simulink model "old_FMS"  (R2018b)
settings: configuration reference "FMS_config" (kept outside this file)
undefined symbols (not defined in the file): actuator_cmd, DiscIntNeverNeededParam, FMS_EXPORT, FMS_PARAM, mode, p_cmd, phi_cmd, psi_rate_cmd, q_cmd, r_cmd, reset, state, theta_cmd, throttle_cmd, timestamp, u_cmd, v_cmd, w_cmd
libraries: simulink x39, Rotation x2, Filter x1
(part 2 of 2)

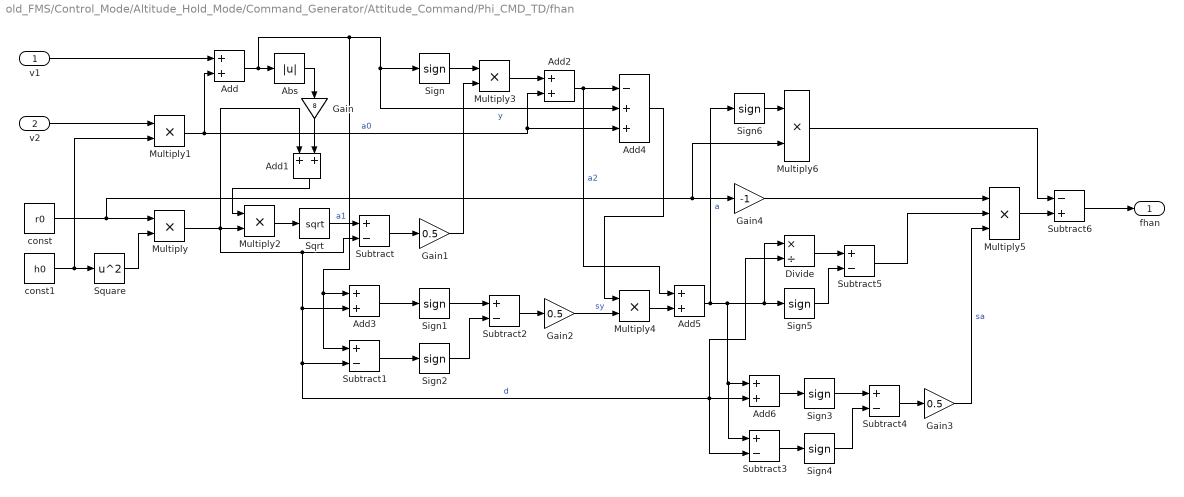
== system old_FMS/Control_Mode/Altitude_Hold_Mode/Command_Generator/Attitude_Command/Phi_CMD_TD/fhan  ==
  v1 : Inport
  v2 : Inport  Port=2
  Abs : Abs
  Add{,1..3,5..6} (6 alike) : Sum  OutDataTypeStr=Inherit: Same as first input
  Add4 : Sum  Inputs=-++
  Divide : Product  Inputs=*/
  Gain : Gain  Gain=8
  Gain1 : Gain  Gain=0.5  OutDataTypeStr=Inherit: Same as input
  Gain2 : Gain  Gain=0.5  OutDataTypeStr=Inherit: Same as input
  Gain3 : Gain  Gain=0.5  OutDataTypeStr=Inherit: Same as input
  Gain4 : Gain  Gain=-1  OutDataTypeStr=Inherit: Same as input
  Multiply{,1..3} (4 alike) : Product  OutDataTypeStr=Inherit: Same as first input
  Multiply4 : Product  OutDataTypeStr=single
  Multiply5 : Product  Inputs=3
  Multiply6 : Product  OutDataTypeStr=single
  Sign{,1..6} (7 alike) : Signum
  Sqrt : Sqrt  SaturateOnIntegerOverflow=on
  Square : Math  Operator=square  SaturateOnIntegerOverflow=on
  Subtract{,1..5} (6 alike) : Sum  Inputs=+-  OutDataTypeStr=Inherit: Same as first input
  Subtract6 : Sum  Inputs=-+  OutDataTypeStr=Inherit: Same as first input
  const : Constant  Value=r0  OutDataTypeStr=single
  const1 : Constant  Value=h0  OutDataTypeStr=single
  fhan : Outport
  wires:
  Sign1/1 -> Subtract2/1
  Multiply2/1 -> Sqrt/1
  Square/1 -> Multiply/2
  Gain1/1 -> Multiply3/2
  Multiply6/1 -> Subtract6/1
  Multiply/1 -> Multiply2/2, Add1/1, Add3/2, Subtract1/2, Add6/2, Subtract3/2, Divide/2, Subtract/2  "d"
  Add6/1 -> Sign3/1
  Sign3/1 -> Subtract4/1
  Sign6/1 -> Multiply6/1
  Multiply5/1 -> Subtract6/2
  Gain4/1 -> Multiply5/1
  Subtract4/1 -> Gain3/1
  Add2/1 -> Add5/1, Add4/1  "a2"
  Subtract2/1 -> Gain2/1
  Add/1 -> Abs/1, Sign/1, Add4/2, Add3/1, Subtract1/1  "y"
  Multiply1/1 -> Add/2, Add2/2, Add4/3  "a0"
  Add5/1 -> Add6/1, Subtract3/1, Divide/1, Sign5/1, Sign6/1  "a"
  const1/1 -> Square/1, Multiply1/2
  Multiply4/1 -> Add5/2
  Subtract5/1 -> Multiply5/2
  Add3/1 -> Sign1/1
  const/1 -> Multiply/1, Gain4/1, Multiply6/2
  Gain/1 -> Add1/2
  Multiply3/1 -> Add2/1
  Divide/1 -> Subtract5/1
  Subtract1/1 -> Sign2/1
  Add1/1 -> Multiply2/1
  Subtract3/1 -> Sign4/1
  Sqrt/1 -> Subtract/1  "a1"
  Sign5/1 -> Subtract5/2
  Add4/1 -> Multiply4/1
  Abs/1 -> Gain/1
  Sign4/1 -> Subtract4/2
  Sign2/1 -> Subtract2/2
  Subtract6/1 -> fhan/1
  Subtract/1 -> Gain1/1
  Gain3/1 -> Multiply5/3  "sa"
  v2/1 -> Multiply1/1
  Gain2/1 -> Multiply4/2  "sy"
  Sign/1 -> Multiply3/1
  v1/1 -> Add/1

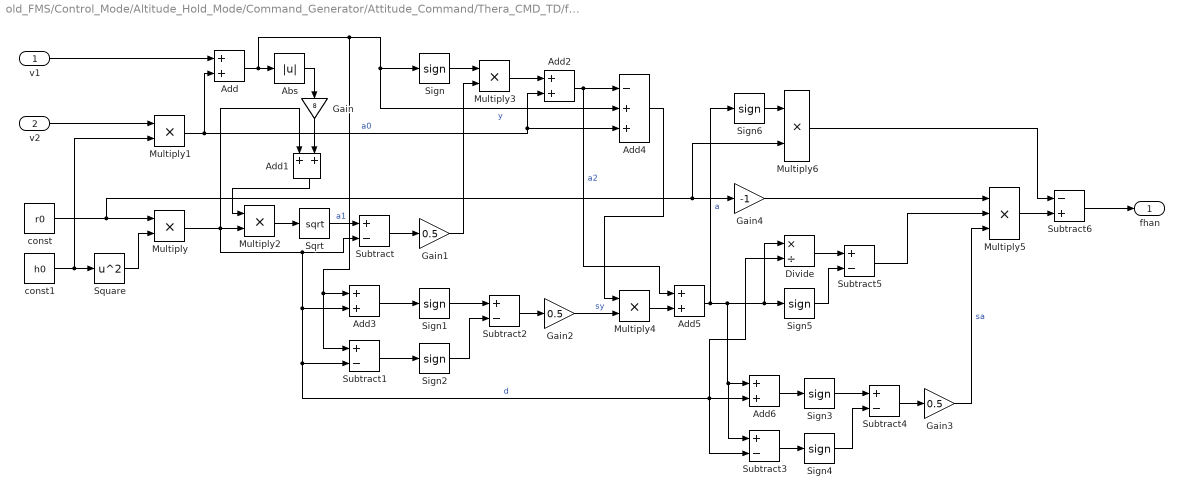
== system old_FMS/Control_Mode/Altitude_Hold_Mode/Command_Generator/Attitude_Command/Thera_CMD_TD/fhan  ==
  v1 : Inport
  v2 : Inport  Port=2
  Abs : Abs
  Add{,1..3,5..6} (6 alike) : Sum  OutDataTypeStr=Inherit: Same as first input
  Add4 : Sum  Inputs=-++
  Divide : Product  Inputs=*/
  Gain : Gain  Gain=8
  Gain1 : Gain  Gain=0.5  OutDataTypeStr=Inherit: Same as input
  Gain2 : Gain  Gain=0.5  OutDataTypeStr=Inherit: Same as input
  Gain3 : Gain  Gain=0.5  OutDataTypeStr=Inherit: Same as input
  Gain4 : Gain  Gain=-1  OutDataTypeStr=Inherit: Same as input
  Multiply{,1..3} (4 alike) : Product  OutDataTypeStr=Inherit: Same as first input
  Multiply4 : Product  OutDataTypeStr=single
  Multiply5 : Product  Inputs=3
  Multiply6 : Product  OutDataTypeStr=single
  Sign{,1..6} (7 alike) : Signum
  Sqrt : Sqrt  SaturateOnIntegerOverflow=on
  Square : Math  Operator=square  SaturateOnIntegerOverflow=on
  Subtract{,1..5} (6 alike) : Sum  Inputs=+-  OutDataTypeStr=Inherit: Same as first input
  Subtract6 : Sum  Inputs=-+  OutDataTypeStr=Inherit: Same as first input
  const : Constant  Value=r0  OutDataTypeStr=single
  const1 : Constant  Value=h0  OutDataTypeStr=single
  fhan : Outport
  wires:
  Sign1/1 -> Subtract2/1
  Multiply2/1 -> Sqrt/1
  Square/1 -> Multiply/2
  Gain1/1 -> Multiply3/2
  Multiply6/1 -> Subtract6/1
  Multiply/1 -> Multiply2/2, Add1/1, Add3/2, Subtract1/2, Add6/2, Subtract3/2, Divide/2, Subtract/2  "d"
  Add6/1 -> Sign3/1
  Sign3/1 -> Subtract4/1
  Sign6/1 -> Multiply6/1
  Multiply5/1 -> Subtract6/2
  Gain4/1 -> Multiply5/1
  Subtract4/1 -> Gain3/1
  Add2/1 -> Add5/1, Add4/1  "a2"
  Subtract2/1 -> Gain2/1
  Add/1 -> Abs/1, Sign/1, Add4/2, Add3/1, Subtract1/1  "y"
  Multiply1/1 -> Add/2, Add2/2, Add4/3  "a0"
  Add5/1 -> Add6/1, Subtract3/1, Divide/1, Sign5/1, Sign6/1  "a"
  const1/1 -> Square/1, Multiply1/2
  Multiply4/1 -> Add5/2
  Subtract5/1 -> Multiply5/2
  Add3/1 -> Sign1/1
  const/1 -> Multiply/1, Gain4/1, Multiply6/2
  Gain/1 -> Add1/2
  Multiply3/1 -> Add2/1
  Divide/1 -> Subtract5/1
  Subtract1/1 -> Sign2/1
  Add1/1 -> Multiply2/1
  Subtract3/1 -> Sign4/1
  Sqrt/1 -> Subtract/1  "a1"
  Sign5/1 -> Subtract5/2
  Add4/1 -> Multiply4/1
  Abs/1 -> Gain/1
  Sign4/1 -> Subtract4/2
  Sign2/1 -> Subtract2/2
  Subtract6/1 -> fhan/1
  Subtract/1 -> Gain1/1
  Gain3/1 -> Multiply5/3  "sa"
  v2/1 -> Multiply1/1
  Gain2/1 -> Multiply4/2  "sy"
  Sign/1 -> Multiply3/1
  v1/1 -> Add/1

== system old_FMS/Control_Mode/Altitude_Hold_Mode/Command_Generator/Psi_Rate_Command/Heading_Control/Heading_Error ==
  INS_Out : Inport
  update : Inport  Port=2
  Bus_Selection : Subsystem
  Holder : Subsystem
  Sum : Sum  Inputs=-+|
  psi_err_rad : Outport
  wires:
  Bus_Selection/1(psi_rad) -> Sum/1, Holder/1(u)
  update/1 -> Holder/2(update)
  INS_Out/1 -> Bus_Selection/1(INS_Out)
  Holder/1(y) -> Sum/2  "psi_hold"
  Sum/1 -> psi_err_rad/1  "psi_err"

== system old_FMS/Control_Mode/Altitude_Hold_Mode/Command_Generator/Psi_Rate_Command/Heading_Rate_Map/Stretch ==
  u : Inport
  Dead Zone : DeadZone  LowerValue=-FMS_PARAM.StickDeadZone  UpperValue=FMS_PARAM.StickDeadZone  SaturateOnIntegerOverflow=on
  Gain : Gain  Gain=1/(1-FMS_PARAM.StickDeadZone)
  y : Outport
  wires:
  u/1 -> Dead Zone/1
  Dead Zone/1 -> Gain/1
  Gain/1 -> y/1

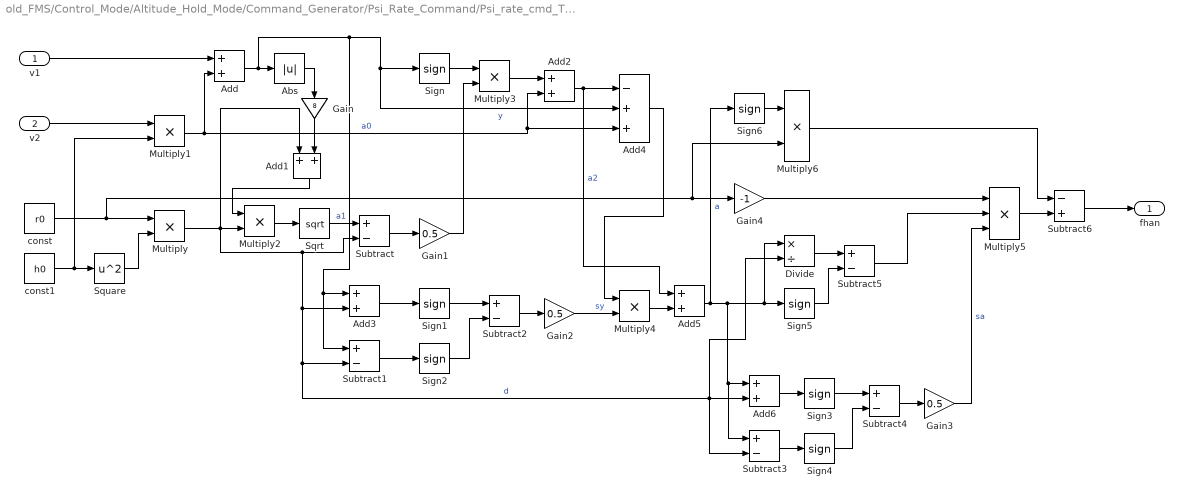
== system old_FMS/Control_Mode/Altitude_Hold_Mode/Command_Generator/Psi_Rate_Command/Psi_rate_cmd_TD/fhan  ==
  v1 : Inport
  v2 : Inport  Port=2
  Abs : Abs
  Add{,1..3,5..6} (6 alike) : Sum  OutDataTypeStr=Inherit: Same as first input
  Add4 : Sum  Inputs=-++
  Divide : Product  Inputs=*/
  Gain : Gain  Gain=8
  Gain1 : Gain  Gain=0.5  OutDataTypeStr=Inherit: Same as input
  Gain2 : Gain  Gain=0.5  OutDataTypeStr=Inherit: Same as input
  Gain3 : Gain  Gain=0.5  OutDataTypeStr=Inherit: Same as input
  Gain4 : Gain  Gain=-1  OutDataTypeStr=Inherit: Same as input
  Multiply{,1..3} (4 alike) : Product  OutDataTypeStr=Inherit: Same as first input
  Multiply4 : Product  OutDataTypeStr=single
  Multiply5 : Product  Inputs=3
  Multiply6 : Product  OutDataTypeStr=single
  Sign{,1..6} (7 alike) : Signum
  Sqrt : Sqrt  SaturateOnIntegerOverflow=on
  Square : Math  Operator=square  SaturateOnIntegerOverflow=on
  Subtract{,1..5} (6 alike) : Sum  Inputs=+-  OutDataTypeStr=Inherit: Same as first input
  Subtract6 : Sum  Inputs=-+  OutDataTypeStr=Inherit: Same as first input
  const : Constant  Value=r0  OutDataTypeStr=single
  const1 : Constant  Value=h0  OutDataTypeStr=single
  fhan : Outport
  wires:
  Sign1/1 -> Subtract2/1
  Multiply2/1 -> Sqrt/1
  Square/1 -> Multiply/2
  Gain1/1 -> Multiply3/2
  Multiply6/1 -> Subtract6/1
  Multiply/1 -> Multiply2/2, Add1/1, Add3/2, Subtract1/2, Add6/2, Subtract3/2, Divide/2, Subtract/2  "d"
  Add6/1 -> Sign3/1
  Sign3/1 -> Subtract4/1
  Sign6/1 -> Multiply6/1
  Multiply5/1 -> Subtract6/2
  Gain4/1 -> Multiply5/1
  Subtract4/1 -> Gain3/1
  Add2/1 -> Add5/1, Add4/1  "a2"
  Subtract2/1 -> Gain2/1
  Add/1 -> Abs/1, Sign/1, Add4/2, Add3/1, Subtract1/1  "y"
  Multiply1/1 -> Add/2, Add2/2, Add4/3  "a0"
  Add5/1 -> Add6/1, Subtract3/1, Divide/1, Sign5/1, Sign6/1  "a"
  const1/1 -> Square/1, Multiply1/2
  Multiply4/1 -> Add5/2
  Subtract5/1 -> Multiply5/2
  Add3/1 -> Sign1/1
  const/1 -> Multiply/1, Gain4/1, Multiply6/2
  Gain/1 -> Add1/2
  Multiply3/1 -> Add2/1
  Divide/1 -> Subtract5/1
  Subtract1/1 -> Sign2/1
  Add1/1 -> Multiply2/1
  Subtract3/1 -> Sign4/1
  Sqrt/1 -> Subtract/1  "a1"
  Sign5/1 -> Subtract5/2
  Add4/1 -> Multiply4/1
  Abs/1 -> Gain/1
  Sign4/1 -> Subtract4/2
  Sign2/1 -> Subtract2/2
  Subtract6/1 -> fhan/1
  Subtract/1 -> Gain1/1
  Gain3/1 -> Multiply5/3  "sa"
  v2/1 -> Multiply1/1
  Gain2/1 -> Multiply4/2  "sy"
  Sign/1 -> Multiply3/1
  v1/1 -> Add/1

== system old_FMS/Control_Mode/Altitude_Hold_Mode/Command_Generator/Vel_Command/Subsystem1/Height_Control ==
  motion_state : Inport
  INS_Out : Inport  Port=2
  Gain4 : Gain  Gain=FMS_PARAM.Z_P  OutDataTypeStr=single
  Position_Error : Subsystem
  vel_w_cmd_C_mPs : Outport
  wires:
  INS_Out/1 -> Position_Error/1(INS_Out)
  Gain4/1 -> vel_w_cmd_C_mPs/1
  Position_Error/1(pos_z_err_R_C) -> Gain4/1
  motion_state/1 -> Position_Error/2(motion_state)

== system old_FMS/Control_Mode/Altitude_Hold_Mode/Command_Generator/Vel_Command/Subsystem1/Velocity_Map ==
  motion_state : Inport
  FMS_Cmd : Inport  Port=2
  Bus Selector1 : BusSelector  OutputSignals=stick_throttle
  Compare To Constant1 : simulink/Logic and Bit Operations/Compare To Constant  relop===  const=1  OutDataTypeStr=boolean
  Constant1 : Constant  Value=0  VectorParams1D=off  OutDataTypeStr=single
  Gain6 : Gain  Gain=-FMS_PARAM.VEL_Z_LIM  OutDataTypeStr=single
  Stretch : Subsystem
  Switch2 : Switch  Criteria=u2 > Threshold
  vel_w_cmd_C_mPs : Outport
  wires:
  Switch2/1 -> vel_w_cmd_C_mPs/1
  Gain6/1 -> Switch2/3
  Bus Selector1/1 -> Stretch/1(u)  "<stick_throttle>"
  Compare To Constant1/1 -> Switch2/2
  motion_state/1 -> Compare To Constant1/1
  Constant1/1 -> Switch2/1  "brake_speed"
  FMS_Cmd/1 -> Bus Selector1/1
  Stretch/1(y) -> Gain6/1

== system old_FMS/Control_Mode/Altitude_Hold_Mode/Command_Generator/Vel_Command/Subsystem1/W_CMD_TD ==
  v : Inport
  Integrator : DiscreteIntegrator  SampleTime=-1  ICPrevOutput=DiscIntNeverNeededParam  ICPrevScaledInput=DiscIntNeverNeededParam
  Integrator1 : DiscreteIntegrator  SampleTime=-1  ICPrevOutput=DiscIntNeverNeededParam  ICPrevScaledInput=DiscIntNeverNeededParam
  Subtract : Sum  Inputs=+-
  "fhan " : Subsystem  mask{r0=4*9.806, h0=0.05}
      mask DialogControl ParameterGroupVar Prompt: fhan(v1,v2,r0,h0)
  v1 : Outport
  wires:
  Integrator1/1 -> v1/1, Subtract/1
  v/1 -> Subtract/2
  Integrator/1 -> "fhan "/2(v2), Integrator1/1  "v2"
  Subtract/1 -> "fhan "/1(v1)
  "fhan "/1(fhan) -> Integrator/1

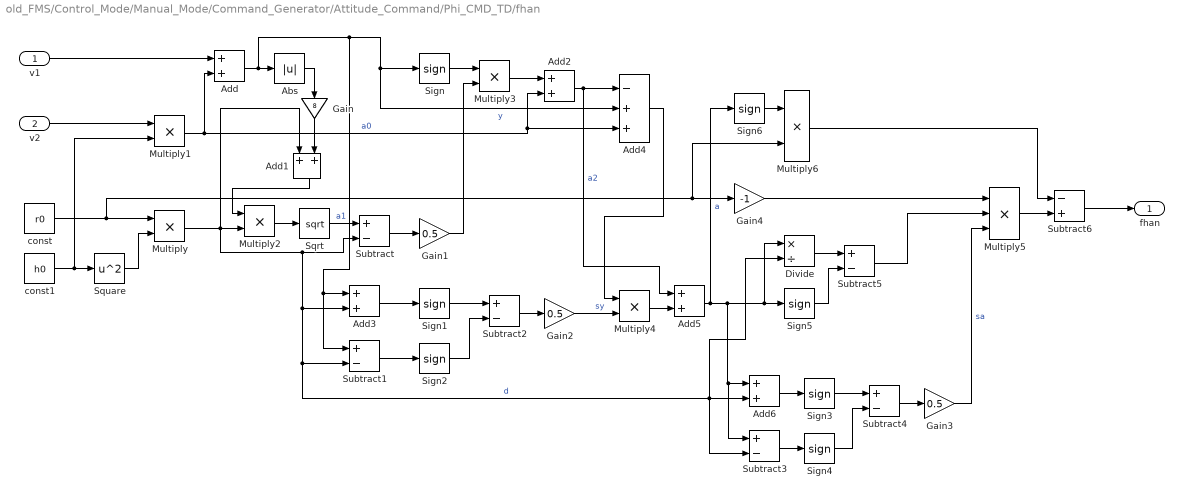
== system old_FMS/Control_Mode/Manual_Mode/Command_Generator/Attitude_Command/Phi_CMD_TD/fhan  ==
  v1 : Inport
  v2 : Inport  Port=2
  Abs : Abs
  Add{,1..3,5..6} (6 alike) : Sum  OutDataTypeStr=Inherit: Same as first input
  Add4 : Sum  Inputs=-++
  Divide : Product  Inputs=*/
  Gain : Gain  Gain=8
  Gain1 : Gain  Gain=0.5  OutDataTypeStr=Inherit: Same as input
  Gain2 : Gain  Gain=0.5  OutDataTypeStr=Inherit: Same as input
  Gain3 : Gain  Gain=0.5  OutDataTypeStr=Inherit: Same as input
  Gain4 : Gain  Gain=-1  OutDataTypeStr=Inherit: Same as input
  Multiply{,1..3} (4 alike) : Product  OutDataTypeStr=Inherit: Same as first input
  Multiply4 : Product  OutDataTypeStr=single
  Multiply5 : Product  Inputs=3
  Multiply6 : Product  OutDataTypeStr=single
  Sign{,1..6} (7 alike) : Signum
  Sqrt : Sqrt  SaturateOnIntegerOverflow=on
  Square : Math  Operator=square  SaturateOnIntegerOverflow=on
  Subtract{,1..5} (6 alike) : Sum  Inputs=+-  OutDataTypeStr=Inherit: Same as first input
  Subtract6 : Sum  Inputs=-+  OutDataTypeStr=Inherit: Same as first input
  const : Constant  Value=r0  OutDataTypeStr=single
  const1 : Constant  Value=h0  OutDataTypeStr=single
  fhan : Outport
  wires:
  Sign1/1 -> Subtract2/1
  Multiply2/1 -> Sqrt/1
  Square/1 -> Multiply/2
  Gain1/1 -> Multiply3/2
  Multiply6/1 -> Subtract6/1
  Multiply/1 -> Multiply2/2, Add1/1, Add3/2, Subtract1/2, Add6/2, Subtract3/2, Divide/2, Subtract/2  "d"
  Add6/1 -> Sign3/1
  Sign3/1 -> Subtract4/1
  Sign6/1 -> Multiply6/1
  Multiply5/1 -> Subtract6/2
  Gain4/1 -> Multiply5/1
  Subtract4/1 -> Gain3/1
  Add2/1 -> Add5/1, Add4/1  "a2"
  Subtract2/1 -> Gain2/1
  Add/1 -> Abs/1, Sign/1, Add4/2, Add3/1, Subtract1/1  "y"
  Multiply1/1 -> Add/2, Add2/2, Add4/3  "a0"
  Add5/1 -> Add6/1, Subtract3/1, Divide/1, Sign5/1, Sign6/1  "a"
  const1/1 -> Square/1, Multiply1/2
  Multiply4/1 -> Add5/2
  Subtract5/1 -> Multiply5/2
  Add3/1 -> Sign1/1
  const/1 -> Multiply/1, Gain4/1, Multiply6/2
  Gain/1 -> Add1/2
  Multiply3/1 -> Add2/1
  Divide/1 -> Subtract5/1
  Subtract1/1 -> Sign2/1
  Add1/1 -> Multiply2/1
  Subtract3/1 -> Sign4/1
  Sqrt/1 -> Subtract/1  "a1"
  Sign5/1 -> Subtract5/2
  Add4/1 -> Multiply4/1
  Abs/1 -> Gain/1
  Sign4/1 -> Subtract4/2
  Sign2/1 -> Subtract2/2
  Subtract6/1 -> fhan/1
  Subtract/1 -> Gain1/1
  Gain3/1 -> Multiply5/3  "sa"
  v2/1 -> Multiply1/1
  Gain2/1 -> Multiply4/2  "sy"
  Sign/1 -> Multiply3/1
  v1/1 -> Add/1

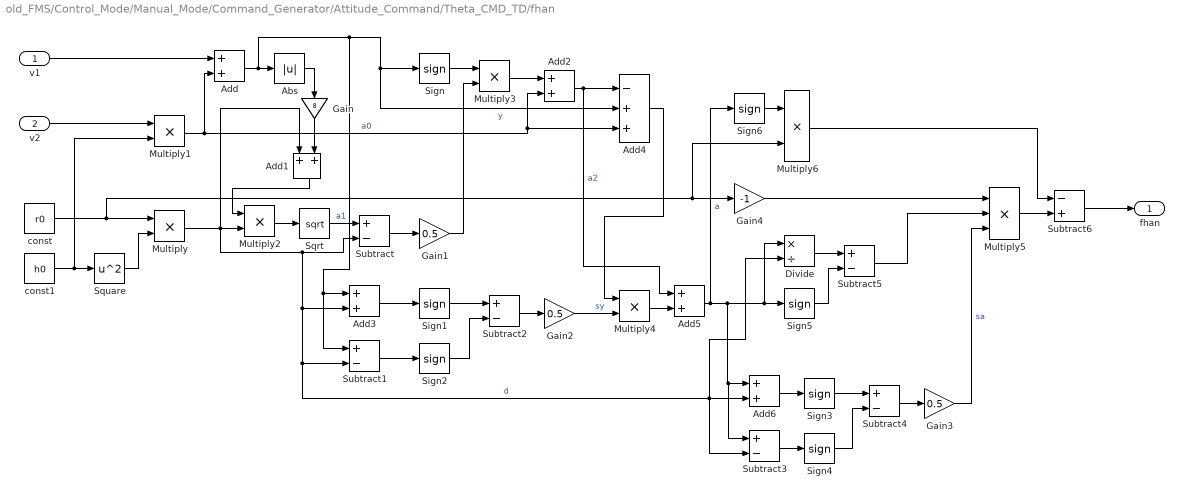
== system old_FMS/Control_Mode/Manual_Mode/Command_Generator/Attitude_Command/Theta_CMD_TD/fhan  ==
  v1 : Inport
  v2 : Inport  Port=2
  Abs : Abs
  Add{,1..3,5..6} (6 alike) : Sum  OutDataTypeStr=Inherit: Same as first input
  Add4 : Sum  Inputs=-++
  Divide : Product  Inputs=*/
  Gain : Gain  Gain=8
  Gain1 : Gain  Gain=0.5  OutDataTypeStr=Inherit: Same as input
  Gain2 : Gain  Gain=0.5  OutDataTypeStr=Inherit: Same as input
  Gain3 : Gain  Gain=0.5  OutDataTypeStr=Inherit: Same as input
  Gain4 : Gain  Gain=-1  OutDataTypeStr=Inherit: Same as input
  Multiply{,1..3} (4 alike) : Product  OutDataTypeStr=Inherit: Same as first input
  Multiply4 : Product  OutDataTypeStr=single
  Multiply5 : Product  Inputs=3
  Multiply6 : Product  OutDataTypeStr=single
  Sign{,1..6} (7 alike) : Signum
  Sqrt : Sqrt  SaturateOnIntegerOverflow=on
  Square : Math  Operator=square  SaturateOnIntegerOverflow=on
  Subtract{,1..5} (6 alike) : Sum  Inputs=+-  OutDataTypeStr=Inherit: Same as first input
  Subtract6 : Sum  Inputs=-+  OutDataTypeStr=Inherit: Same as first input
  const : Constant  Value=r0  OutDataTypeStr=single
  const1 : Constant  Value=h0  OutDataTypeStr=single
  fhan : Outport
  wires:
  Sign1/1 -> Subtract2/1
  Multiply2/1 -> Sqrt/1
  Square/1 -> Multiply/2
  Gain1/1 -> Multiply3/2
  Multiply6/1 -> Subtract6/1
  Multiply/1 -> Multiply2/2, Add1/1, Add3/2, Subtract1/2, Add6/2, Subtract3/2, Divide/2, Subtract/2  "d"
  Add6/1 -> Sign3/1
  Sign3/1 -> Subtract4/1
  Sign6/1 -> Multiply6/1
  Multiply5/1 -> Subtract6/2
  Gain4/1 -> Multiply5/1
  Subtract4/1 -> Gain3/1
  Add2/1 -> Add5/1, Add4/1  "a2"
  Subtract2/1 -> Gain2/1
  Add/1 -> Abs/1, Sign/1, Add4/2, Add3/1, Subtract1/1  "y"
  Multiply1/1 -> Add/2, Add2/2, Add4/3  "a0"
  Add5/1 -> Add6/1, Subtract3/1, Divide/1, Sign5/1, Sign6/1  "a"
  const1/1 -> Square/1, Multiply1/2
  Multiply4/1 -> Add5/2
  Subtract5/1 -> Multiply5/2
  Add3/1 -> Sign1/1
  const/1 -> Multiply/1, Gain4/1, Multiply6/2
  Gain/1 -> Add1/2
  Multiply3/1 -> Add2/1
  Divide/1 -> Subtract5/1
  Subtract1/1 -> Sign2/1
  Add1/1 -> Multiply2/1
  Subtract3/1 -> Sign4/1
  Sqrt/1 -> Subtract/1  "a1"
  Sign5/1 -> Subtract5/2
  Add4/1 -> Multiply4/1
  Abs/1 -> Gain/1
  Sign4/1 -> Subtract4/2
  Sign2/1 -> Subtract2/2
  Subtract6/1 -> fhan/1
  Subtract/1 -> Gain1/1
  Gain3/1 -> Multiply5/3  "sa"
  v2/1 -> Multiply1/1
  Gain2/1 -> Multiply4/2  "sy"
  Sign/1 -> Multiply3/1
  v1/1 -> Add/1

== system old_FMS/Control_Mode/Manual_Mode/Command_Generator/Psi_Rate_Command/Heading_Control/Heading_Error ==
  INS_Out : Inport
  update : Inport  Port=2
  Bus_Selection : Subsystem
  Holder : Subsystem
  Sum : Sum  Inputs=-+|
  psi_err_rad : Outport
  wires:
  Sum/1 -> psi_err_rad/1
  Holder/1(y) -> Sum/2
  INS_Out/1 -> Bus_Selection/1(INS_Out)
  update/1 -> Holder/2(update)
  Bus_Selection/1(psi_rad) -> Holder/1(u), Sum/1

== system old_FMS/Control_Mode/Manual_Mode/Command_Generator/Psi_Rate_Command/Heading_Rate_Map/Stretch ==
  u : Inport
  Dead Zone : DeadZone  LowerValue=-FMS_PARAM.StickDeadZone  UpperValue=FMS_PARAM.StickDeadZone  SaturateOnIntegerOverflow=on
  Gain : Gain  Gain=1/(1-FMS_PARAM.StickDeadZone)
  y : Outport
  wires:
  Gain/1 -> y/1
  Dead Zone/1 -> Gain/1
  u/1 -> Dead Zone/1

== system old_FMS/Control_Mode/Position_Mode/Command_Generator/Psi_Rate_Command1/Heading_Control/Heading_Error ==
  INS_Out : Inport
  update : Inport  Port=2
  Bus_Selection : Subsystem
  Holder : Subsystem
  Sum : Sum  Inputs=-+|
  psi_err_rad : Outport
  wires:
  Bus_Selection/1(psi_rad) -> Sum/1, Holder/1(u)
  update/1 -> Holder/2(update)
  INS_Out/1 -> Bus_Selection/1(INS_Out)
  Holder/1(y) -> Sum/2  "psi_hold"
  Sum/1 -> psi_err_rad/1  "psi_err"

== system old_FMS/Control_Mode/Position_Mode/Command_Generator/Psi_Rate_Command1/Heading_Rate_Map/Stretch ==
  u : Inport
  Dead Zone : DeadZone  LowerValue=-FMS_PARAM.StickDeadZone  UpperValue=FMS_PARAM.StickDeadZone  SaturateOnIntegerOverflow=on
  Gain : Gain  Gain=1/(1-FMS_PARAM.StickDeadZone)
  y : Outport
  wires:
  u/1 -> Dead Zone/1
  Dead Zone/1 -> Gain/1
  Gain/1 -> y/1

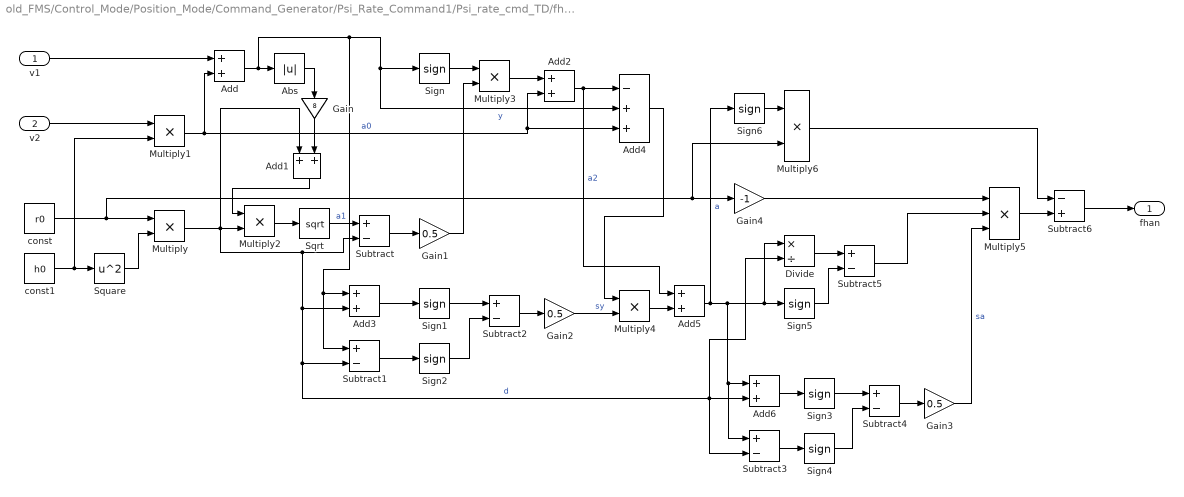
== system old_FMS/Control_Mode/Position_Mode/Command_Generator/Psi_Rate_Command1/Psi_rate_cmd_TD/fhan  ==
  v1 : Inport
  v2 : Inport  Port=2
  Abs : Abs
  Add{,1..3,5..6} (6 alike) : Sum  OutDataTypeStr=Inherit: Same as first input
  Add4 : Sum  Inputs=-++
  Divide : Product  Inputs=*/
  Gain : Gain  Gain=8
  Gain1 : Gain  Gain=0.5  OutDataTypeStr=Inherit: Same as input
  Gain2 : Gain  Gain=0.5  OutDataTypeStr=Inherit: Same as input
  Gain3 : Gain  Gain=0.5  OutDataTypeStr=Inherit: Same as input
  Gain4 : Gain  Gain=-1  OutDataTypeStr=Inherit: Same as input
  Multiply{,1..3} (4 alike) : Product  OutDataTypeStr=Inherit: Same as first input
  Multiply4 : Product  OutDataTypeStr=single
  Multiply5 : Product  Inputs=3
  Multiply6 : Product  OutDataTypeStr=single
  Sign{,1..6} (7 alike) : Signum
  Sqrt : Sqrt  SaturateOnIntegerOverflow=on
  Square : Math  Operator=square  SaturateOnIntegerOverflow=on
  Subtract{,1..5} (6 alike) : Sum  Inputs=+-  OutDataTypeStr=Inherit: Same as first input
  Subtract6 : Sum  Inputs=-+  OutDataTypeStr=Inherit: Same as first input
  const : Constant  Value=r0  OutDataTypeStr=single
  const1 : Constant  Value=h0  OutDataTypeStr=single
  fhan : Outport
  wires:
  Sign1/1 -> Subtract2/1
  Multiply2/1 -> Sqrt/1
  Square/1 -> Multiply/2
  Gain1/1 -> Multiply3/2
  Multiply6/1 -> Subtract6/1
  Multiply/1 -> Multiply2/2, Add1/1, Add3/2, Subtract1/2, Add6/2, Subtract3/2, Divide/2, Subtract/2  "d"
  Add6/1 -> Sign3/1
  Sign3/1 -> Subtract4/1
  Sign6/1 -> Multiply6/1
  Multiply5/1 -> Subtract6/2
  Gain4/1 -> Multiply5/1
  Subtract4/1 -> Gain3/1
  Add2/1 -> Add5/1, Add4/1  "a2"
  Subtract2/1 -> Gain2/1
  Add/1 -> Abs/1, Sign/1, Add4/2, Add3/1, Subtract1/1  "y"
  Multiply1/1 -> Add/2, Add2/2, Add4/3  "a0"
  Add5/1 -> Add6/1, Subtract3/1, Divide/1, Sign5/1, Sign6/1  "a"
  const1/1 -> Square/1, Multiply1/2
  Multiply4/1 -> Add5/2
  Subtract5/1 -> Multiply5/2
  Add3/1 -> Sign1/1
  const/1 -> Multiply/1, Gain4/1, Multiply6/2
  Gain/1 -> Add1/2
  Multiply3/1 -> Add2/1
  Divide/1 -> Subtract5/1
  Subtract1/1 -> Sign2/1
  Add1/1 -> Multiply2/1
  Subtract3/1 -> Sign4/1
  Sqrt/1 -> Subtract/1  "a1"
  Sign5/1 -> Subtract5/2
  Add4/1 -> Multiply4/1
  Abs/1 -> Gain/1
  Sign4/1 -> Subtract4/2
  Sign2/1 -> Subtract2/2
  Subtract6/1 -> fhan/1
  Subtract/1 -> Gain1/1
  Gain3/1 -> Multiply5/3  "sa"
  v2/1 -> Multiply1/1
  Gain2/1 -> Multiply4/2  "sy"
  Sign/1 -> Multiply3/1
  v1/1 -> Add/1

== system old_FMS/Control_Mode/Position_Mode/Command_Generator/Vel_Command/Subsystem1/Position_Control ==
  M_CO : Inport
  motion_state : Inport  Port=2
  INS_Out : Inport  Port=3
  Gain2 : Gain  Gain=FMS_PARAM.XY_P  OutDataTypeStr=single
  Gain4 : Gain  Gain=FMS_PARAM.Z_P  OutDataTypeStr=single
  Position_Error : Subsystem
  Selector : Selector  InputPortWidth=3  IndexOptions=Index vector (dialog)  Indices=3  OutputSizes=1
  Selector1 : Selector  InputPortWidth=3  IndexOptions=Index vector (dialog)  Indices=[1 2]  OutputSizes=1
  vel_uv_cmd_C_mPs : Outport
  vel_w_cmd_C_mPs : Outport  Port=2
  wires:
  INS_Out/1 -> Position_Error/2(INS_Out)
  Gain4/1 -> vel_w_cmd_C_mPs/1
  Gain2/1 -> vel_uv_cmd_C_mPs/1
  M_CO/1 -> Position_Error/1(M_CO)
  motion_state/1 -> Position_Error/3(motion_state)
  Position_Error/1(pos_err_R_C) -> Selector/1, Selector1/1
  Selector1/1 -> Gain2/1
  Selector/1 -> Gain4/1

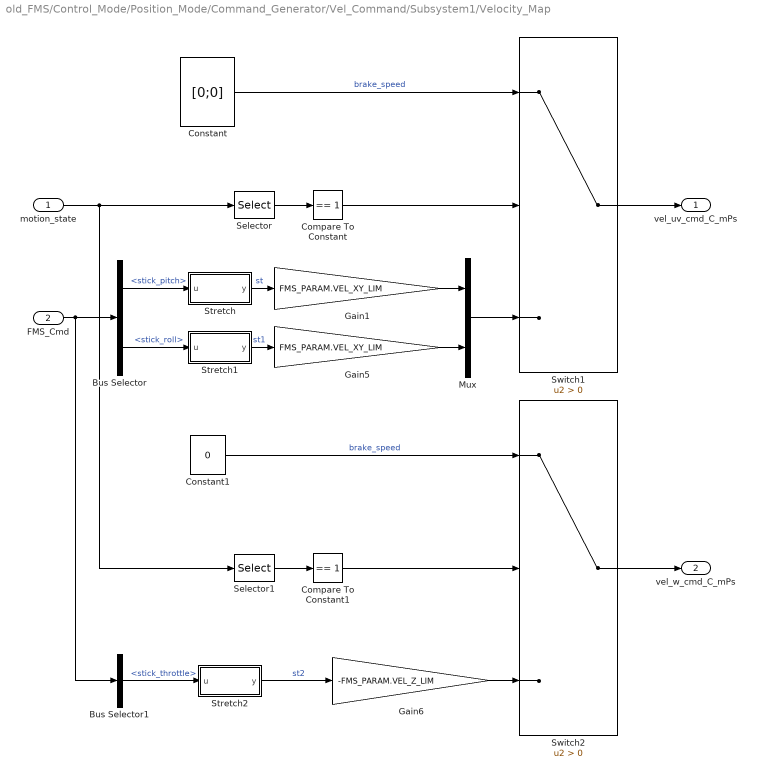
== system old_FMS/Control_Mode/Position_Mode/Command_Generator/Vel_Command/Subsystem1/Velocity_Map ==
  motion_state : Inport
  FMS_Cmd : Inport  Port=2
  Bus Selector : BusSelector  OutputSignals=stick_pitch,stick_roll
  Bus Selector1 : BusSelector  OutputSignals=stick_throttle
  Compare To Constant : simulink/Logic and Bit Operations/Compare To Constant  relop===  const=1  OutDataTypeStr=boolean
  Compare To Constant1 : simulink/Logic and Bit Operations/Compare To Constant  relop===  const=1  OutDataTypeStr=boolean
  Constant : Constant  Value=[0;0]  VectorParams1D=off  OutDataTypeStr=single
  Constant1 : Constant  Value=0  VectorParams1D=off  OutDataTypeStr=single
  Gain1 : Gain  Gain=FMS_PARAM.VEL_XY_LIM  OutDataTypeStr=single
  Gain5 : Gain  Gain=FMS_PARAM.VEL_XY_LIM  OutDataTypeStr=single
  Gain6 : Gain  Gain=-FMS_PARAM.VEL_Z_LIM  OutDataTypeStr=single
  Mux : Mux  Inputs=2
  Selector : Selector  InputPortWidth=2  IndexOptions=Index vector (dialog)  Indices=1  OutputSizes=1
  Selector1 : Selector  InputPortWidth=2  IndexOptions=Index vector (dialog)  Indices=2  OutputSizes=1
  Stretch : Subsystem
  Stretch1 : Subsystem
  Stretch2 : Subsystem
  Switch1 : Switch  Criteria=u2 > Threshold
  Switch2 : Switch  Criteria=u2 > Threshold
  vel_uv_cmd_C_mPs : Outport
  vel_w_cmd_C_mPs : Outport  Port=2
  wires:
  Switch2/1 -> vel_w_cmd_C_mPs/1
  Gain6/1 -> Switch2/3
  Bus Selector1/1 -> Stretch2/1(u)  "<stick_throttle>"
  motion_state/1 -> Selector/1, Selector1/1
  Compare To Constant1/1 -> Switch2/2
  Selector1/1 -> Compare To Constant1/1
  Constant1/1 -> Switch2/1  "brake_speed"
  FMS_Cmd/1 -> Bus Selector/1, Bus Selector1/1
  Selector/1 -> Compare To Constant/1
  Bus Selector/1 -> Stretch/1(u)  "<stick_pitch>"
  Compare To Constant/1 -> Switch1/2
  Gain1/1 -> Mux/1
  Bus Selector/2 -> Stretch1/1(u)  "<stick_roll>"
  Gain5/1 -> Mux/2
  Switch1/1 -> vel_uv_cmd_C_mPs/1
  Mux/1 -> Switch1/3
  Constant/1 -> Switch1/1  "brake_speed"
  Stretch/1(y) -> Gain1/1  "st"
  Stretch1/1(y) -> Gain5/1  "st1"
  Stretch2/1(y) -> Gain6/1  "st2"

== system old_FMS/Control_Mode/Position_Mode/Command_Generator/Vel_Command/Subsystem1/W_CMD_TD ==
  v : Inport
  Integrator : DiscreteIntegrator  SampleTime=-1  ICPrevOutput=DiscIntNeverNeededParam  ICPrevScaledInput=DiscIntNeverNeededParam
  Integrator1 : DiscreteIntegrator  SampleTime=-1  ICPrevOutput=DiscIntNeverNeededParam  ICPrevScaledInput=DiscIntNeverNeededParam
  Subtract : Sum  Inputs=+-
  "fhan " : Subsystem  mask{r0=4*9.806, h0=0.05}
      mask DialogControl ParameterGroupVar Prompt: fhan(v1,v2,r0,h0)
  v1 : Outport
  wires:
  Integrator1/1 -> v1/1, Subtract/1
  v/1 -> Subtract/2
  Integrator/1 -> "fhan "/2(v2), Integrator1/1  "v2"
  Subtract/1 -> "fhan "/1(v1)
  "fhan "/1(fhan) -> Integrator/1

== system old_FMS/Control_Mode/Altitude_Hold_Mode/Command_Generator/Psi_Rate_Command/Heading_Control/Heading_Error/Bus_Selection ==
  INS_Out : Inport
  Bus Selector2 : BusSelector  OutputSignals=psi
  psi_rad : Outport
  wires:
  INS_Out/1 -> Bus Selector2/1
  Bus Selector2/1 -> psi_rad/1  "<psi>"

== system old_FMS/Control_Mode/Altitude_Hold_Mode/Command_Generator/Psi_Rate_Command/Heading_Control/Heading_Error/Holder ==
  u : Inport
  update : Inport  Port=2
  Delay : Delay  DelayLength=1  InitialConditionSource=Input port
      settings: InputPortMap=u0,p4
  Switch1 : Switch  Criteria=u2 > Threshold
  y : Outport
  wires:
  Switch1/1 -> y/1, Delay/1
  Delay/1 -> Switch1/3
  update/1 -> Switch1/2
  u/1 -> Delay/2, Switch1/1

== system old_FMS/Control_Mode/Altitude_Hold_Mode/Command_Generator/Vel_Command/Subsystem1/Height_Control/Position_Error ==
  INS_Out : Inport
  motion_state : Inport  Port=2
  Bus_Selection : Subsystem
  Compare To Constant1 : simulink/Logic and Bit Operations/Compare To Constant  relop===  const=2  OutDataTypeStr=boolean
  Detect Increase1 : simulink/Logic and Bit Operations/Detect Increase  vinit=0.0  OutDataTypeStr=boolean
  Sum : Sum  Inputs=-+|
  Z_Holder : Subsystem
  pos_z_err_R_C : Outport
  wires:
  Z_Holder/1(y) -> Sum/2  "hold_z"
  Detect Increase1/1 -> Z_Holder/2(update)
  Compare To Constant1/1 -> Detect Increase1/1
  motion_state/1 -> Compare To Constant1/1
  Sum/1 -> pos_z_err_R_C/1
  INS_Out/1 -> Bus_Selection/1(INS_Out)
  Bus_Selection/1(pos_z_O) -> Sum/1, Z_Holder/1(u)  "pos_z"

== system old_FMS/Control_Mode/Altitude_Hold_Mode/Command_Generator/Vel_Command/Subsystem1/Velocity_Map/Stretch ==
  u : Inport
  Dead Zone : DeadZone  LowerValue=-FMS_PARAM.StickDeadZone  UpperValue=FMS_PARAM.StickDeadZone  SaturateOnIntegerOverflow=on
  Gain : Gain  Gain=1/(1-FMS_PARAM.StickDeadZone)
  y : Outport
  wires:
  u/1 -> Dead Zone/1
  Dead Zone/1 -> Gain/1
  Gain/1 -> y/1

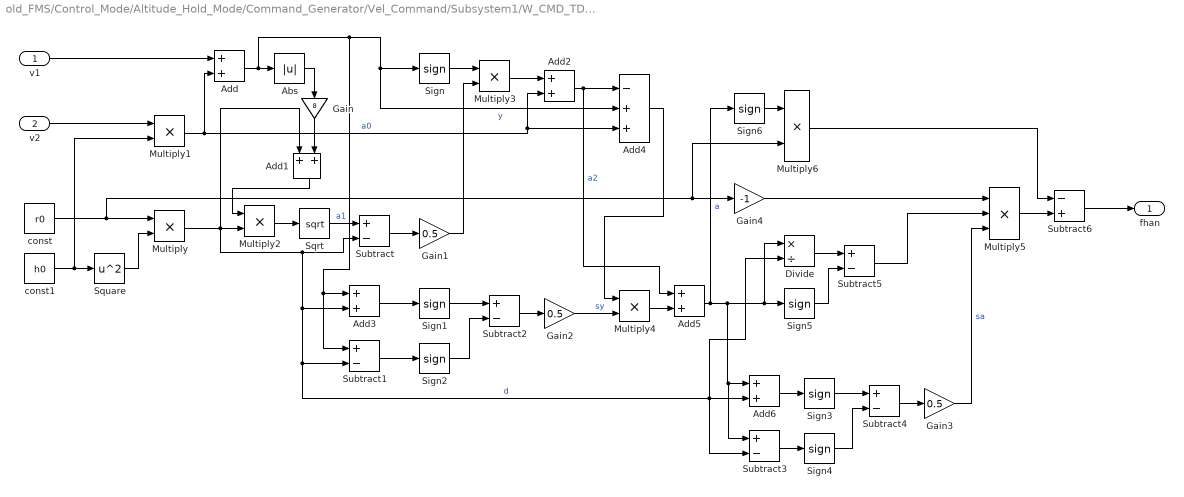
== system old_FMS/Control_Mode/Altitude_Hold_Mode/Command_Generator/Vel_Command/Subsystem1/W_CMD_TD/fhan  ==
  v1 : Inport
  v2 : Inport  Port=2
  Abs : Abs
  Add{,1..3,5..6} (6 alike) : Sum  OutDataTypeStr=Inherit: Same as first input
  Add4 : Sum  Inputs=-++
  Divide : Product  Inputs=*/
  Gain : Gain  Gain=8
  Gain1 : Gain  Gain=0.5  OutDataTypeStr=Inherit: Same as input
  Gain2 : Gain  Gain=0.5  OutDataTypeStr=Inherit: Same as input
  Gain3 : Gain  Gain=0.5  OutDataTypeStr=Inherit: Same as input
  Gain4 : Gain  Gain=-1  OutDataTypeStr=Inherit: Same as input
  Multiply{,1..3} (4 alike) : Product  OutDataTypeStr=Inherit: Same as first input
  Multiply4 : Product  OutDataTypeStr=single
  Multiply5 : Product  Inputs=3
  Multiply6 : Product  OutDataTypeStr=single
  Sign{,1..6} (7 alike) : Signum
  Sqrt : Sqrt  SaturateOnIntegerOverflow=on
  Square : Math  Operator=square  SaturateOnIntegerOverflow=on
  Subtract{,1..5} (6 alike) : Sum  Inputs=+-  OutDataTypeStr=Inherit: Same as first input
  Subtract6 : Sum  Inputs=-+  OutDataTypeStr=Inherit: Same as first input
  const : Constant  Value=r0  OutDataTypeStr=single
  const1 : Constant  Value=h0  OutDataTypeStr=single
  fhan : Outport
  wires:
  Sign1/1 -> Subtract2/1
  Multiply2/1 -> Sqrt/1
  Square/1 -> Multiply/2
  Gain1/1 -> Multiply3/2
  Multiply6/1 -> Subtract6/1
  Multiply/1 -> Multiply2/2, Add1/1, Add3/2, Subtract1/2, Add6/2, Subtract3/2, Divide/2, Subtract/2  "d"
  Add6/1 -> Sign3/1
  Sign3/1 -> Subtract4/1
  Sign6/1 -> Multiply6/1
  Multiply5/1 -> Subtract6/2
  Gain4/1 -> Multiply5/1
  Subtract4/1 -> Gain3/1
  Add2/1 -> Add5/1, Add4/1  "a2"
  Subtract2/1 -> Gain2/1
  Add/1 -> Abs/1, Sign/1, Add4/2, Add3/1, Subtract1/1  "y"
  Multiply1/1 -> Add/2, Add2/2, Add4/3  "a0"
  Add5/1 -> Add6/1, Subtract3/1, Divide/1, Sign5/1, Sign6/1  "a"
  const1/1 -> Square/1, Multiply1/2
  Multiply4/1 -> Add5/2
  Subtract5/1 -> Multiply5/2
  Add3/1 -> Sign1/1
  const/1 -> Multiply/1, Gain4/1, Multiply6/2
  Gain/1 -> Add1/2
  Multiply3/1 -> Add2/1
  Divide/1 -> Subtract5/1
  Subtract1/1 -> Sign2/1
  Add1/1 -> Multiply2/1
  Subtract3/1 -> Sign4/1
  Sqrt/1 -> Subtract/1  "a1"
  Sign5/1 -> Subtract5/2
  Add4/1 -> Multiply4/1
  Abs/1 -> Gain/1
  Sign4/1 -> Subtract4/2
  Sign2/1 -> Subtract2/2
  Subtract6/1 -> fhan/1
  Subtract/1 -> Gain1/1
  Gain3/1 -> Multiply5/3  "sa"
  v2/1 -> Multiply1/1
  Gain2/1 -> Multiply4/2  "sy"
  Sign/1 -> Multiply3/1
  v1/1 -> Add/1

== system old_FMS/Control_Mode/Manual_Mode/Command_Generator/Psi_Rate_Command/Heading_Control/Heading_Error/Bus_Selection ==
  INS_Out : Inport
  Bus Selector2 : BusSelector  OutputSignals=psi
  psi_rad : Outport
  wires:
  Bus Selector2/1 -> psi_rad/1  "<psi>"
  INS_Out/1 -> Bus Selector2/1

== system old_FMS/Control_Mode/Manual_Mode/Command_Generator/Psi_Rate_Command/Heading_Control/Heading_Error/Holder ==
  u : Inport
  update : Inport  Port=2
  Delay : Delay  DelayLength=1  InitialConditionSource=Input port
      settings: InputPortMap=u0,p4
  Switch1 : Switch  Criteria=u2 > Threshold
  y : Outport
  wires:
  u/1 -> Delay/2, Switch1/1
  update/1 -> Switch1/2
  Delay/1 -> Switch1/3
  Switch1/1 -> Delay/1, y/1

== system old_FMS/Control_Mode/Position_Mode/Command_Generator/Psi_Rate_Command1/Heading_Control/Heading_Error/Bus_Selection ==
  INS_Out : Inport
  Bus Selector2 : BusSelector  OutputSignals=psi
  psi_rad : Outport
  wires:
  INS_Out/1 -> Bus Selector2/1
  Bus Selector2/1 -> psi_rad/1  "<psi>"

== system old_FMS/Control_Mode/Position_Mode/Command_Generator/Psi_Rate_Command1/Heading_Control/Heading_Error/Holder ==
  u : Inport
  update : Inport  Port=2
  Delay : Delay  DelayLength=1  InitialConditionSource=Input port
      settings: InputPortMap=u0,p4
  Switch1 : Switch  Criteria=u2 > Threshold
  y : Outport
  wires:
  Switch1/1 -> y/1, Delay/1
  Delay/1 -> Switch1/3
  update/1 -> Switch1/2
  u/1 -> Delay/2, Switch1/1

== system old_FMS/Control_Mode/Position_Mode/Command_Generator/Vel_Command/Subsystem1/Position_Control/Position_Error ==
  M_CO : Inport
  INS_Out : Inport  Port=2
  motion_state : Inport  Port=3
  Bus_Selection : Subsystem
  Compare To Constant : simulink/Logic and Bit Operations/Compare To Constant  relop===  const=2  OutDataTypeStr=boolean
  Compare To Constant1 : simulink/Logic and Bit Operations/Compare To Constant  relop===  const=2  OutDataTypeStr=boolean
  Detect Increase : simulink/Logic and Bit Operations/Detect Increase  vinit=0.0  OutDataTypeStr=boolean
  Detect Increase1 : simulink/Logic and Bit Operations/Detect Increase  vinit=0.0  OutDataTypeStr=boolean
  Multiply : Product  Multiplication=Matrix(*)
  Mux : Mux  Inputs=2
  Selector : Selector  InputPortWidth=2  IndexOptions=Index vector (dialog)  Indices=1  OutputSizes=1
  Selector1 : Selector  InputPortWidth=2  IndexOptions=Index vector (dialog)  Indices=2  OutputSizes=1
  Selector2 : Selector  InputPortWidth=3  IndexOptions=Index vector (dialog)  Indices=[1 2]  OutputSizes=1
  Selector3 : Selector  InputPortWidth=3  IndexOptions=Index vector (dialog)  Indices=3  OutputSizes=1
  Sum : Sum  Inputs=-+|
  XY_Holder : Subsystem
  Z_Holder : Subsystem
  pos_err_R_C : Outport
  wires:
  Mux/1 -> Sum/2  "pos_hold"
  Z_Holder/1(y) -> Mux/2
  Selector3/1 -> Z_Holder/1(u)
  Selector2/1 -> XY_Holder/1(u)
  Detect Increase1/1 -> Z_Holder/2(update)
  Compare To Constant1/1 -> Detect Increase1/1
  Detect Increase/1 -> XY_Holder/2(update)
  Selector1/1 -> Compare To Constant1/1
  Compare To Constant/1 -> Detect Increase/1
  Selector/1 -> Compare To Constant/1
  M_CO/1 -> Multiply/1
  Multiply/1 -> pos_err_R_C/1
  XY_Holder/1(y) -> Mux/1
  INS_Out/1 -> Bus_Selection/1(INS_Out)
  motion_state/1 -> Selector/1, Selector1/1
  Sum/1 -> Multiply/2
  Bus_Selection/1(pos_R_O) -> Selector2/1, Selector3/1, Sum/1  "pos_est"

== system old_FMS/Control_Mode/Position_Mode/Command_Generator/Vel_Command/Subsystem1/Velocity_Map/Stretch ==
  u : Inport
  Dead Zone : DeadZone  LowerValue=-FMS_PARAM.StickDeadZone  UpperValue=FMS_PARAM.StickDeadZone  SaturateOnIntegerOverflow=on
  Gain : Gain  Gain=1/(1-FMS_PARAM.StickDeadZone)
  y : Outport
  wires:
  u/1 -> Dead Zone/1
  Dead Zone/1 -> Gain/1
  Gain/1 -> y/1

== system old_FMS/Control_Mode/Position_Mode/Command_Generator/Vel_Command/Subsystem1/Velocity_Map/Stretch1 ==
  u : Inport
  Dead Zone : DeadZone  LowerValue=-FMS_PARAM.StickDeadZone  UpperValue=FMS_PARAM.StickDeadZone  SaturateOnIntegerOverflow=on
  Gain : Gain  Gain=1/(1-FMS_PARAM.StickDeadZone)
  y : Outport
  wires:
  Gain/1 -> y/1
  Dead Zone/1 -> Gain/1
  u/1 -> Dead Zone/1

== system old_FMS/Control_Mode/Position_Mode/Command_Generator/Vel_Command/Subsystem1/Velocity_Map/Stretch2 ==
  u : Inport
  Dead Zone : DeadZone  LowerValue=-FMS_PARAM.StickDeadZone  UpperValue=FMS_PARAM.StickDeadZone  SaturateOnIntegerOverflow=on
  Gain : Gain  Gain=1/(1-FMS_PARAM.StickDeadZone)
  y : Outport
  wires:
  Gain/1 -> y/1
  Dead Zone/1 -> Gain/1
  u/1 -> Dead Zone/1

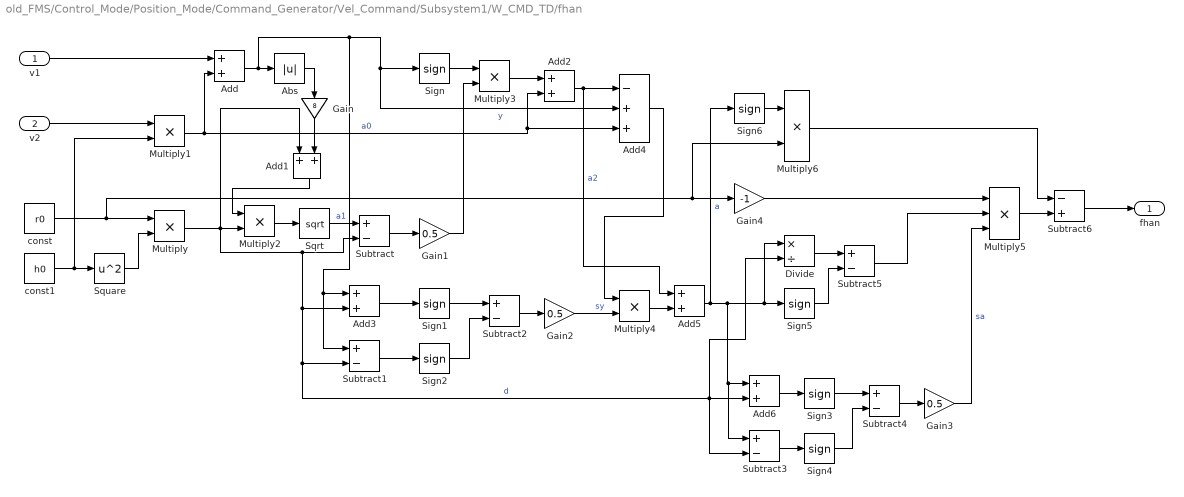
== system old_FMS/Control_Mode/Position_Mode/Command_Generator/Vel_Command/Subsystem1/W_CMD_TD/fhan  ==
  v1 : Inport
  v2 : Inport  Port=2
  Abs : Abs
  Add{,1..3,5..6} (6 alike) : Sum  OutDataTypeStr=Inherit: Same as first input
  Add4 : Sum  Inputs=-++
  Divide : Product  Inputs=*/
  Gain : Gain  Gain=8
  Gain1 : Gain  Gain=0.5  OutDataTypeStr=Inherit: Same as input
  Gain2 : Gain  Gain=0.5  OutDataTypeStr=Inherit: Same as input
  Gain3 : Gain  Gain=0.5  OutDataTypeStr=Inherit: Same as input
  Gain4 : Gain  Gain=-1  OutDataTypeStr=Inherit: Same as input
  Multiply{,1..3} (4 alike) : Product  OutDataTypeStr=Inherit: Same as first input
  Multiply4 : Product  OutDataTypeStr=single
  Multiply5 : Product  Inputs=3
  Multiply6 : Product  OutDataTypeStr=single
  Sign{,1..6} (7 alike) : Signum
  Sqrt : Sqrt  SaturateOnIntegerOverflow=on
  Square : Math  Operator=square  SaturateOnIntegerOverflow=on
  Subtract{,1..5} (6 alike) : Sum  Inputs=+-  OutDataTypeStr=Inherit: Same as first input
  Subtract6 : Sum  Inputs=-+  OutDataTypeStr=Inherit: Same as first input
  const : Constant  Value=r0  OutDataTypeStr=single
  const1 : Constant  Value=h0  OutDataTypeStr=single
  fhan : Outport
  wires:
  Sign1/1 -> Subtract2/1
  Multiply2/1 -> Sqrt/1
  Square/1 -> Multiply/2
  Gain1/1 -> Multiply3/2
  Multiply6/1 -> Subtract6/1
  Multiply/1 -> Multiply2/2, Add1/1, Add3/2, Subtract1/2, Add6/2, Subtract3/2, Divide/2, Subtract/2  "d"
  Add6/1 -> Sign3/1
  Sign3/1 -> Subtract4/1
  Sign6/1 -> Multiply6/1
  Multiply5/1 -> Subtract6/2
  Gain4/1 -> Multiply5/1
  Subtract4/1 -> Gain3/1
  Add2/1 -> Add5/1, Add4/1  "a2"
  Subtract2/1 -> Gain2/1
  Add/1 -> Abs/1, Sign/1, Add4/2, Add3/1, Subtract1/1  "y"
  Multiply1/1 -> Add/2, Add2/2, Add4/3  "a0"
  Add5/1 -> Add6/1, Subtract3/1, Divide/1, Sign5/1, Sign6/1  "a"
  const1/1 -> Square/1, Multiply1/2
  Multiply4/1 -> Add5/2
  Subtract5/1 -> Multiply5/2
  Add3/1 -> Sign1/1
  const/1 -> Multiply/1, Gain4/1, Multiply6/2
  Gain/1 -> Add1/2
  Multiply3/1 -> Add2/1
  Divide/1 -> Subtract5/1
  Subtract1/1 -> Sign2/1
  Add1/1 -> Multiply2/1
  Subtract3/1 -> Sign4/1
  Sqrt/1 -> Subtract/1  "a1"
  Sign5/1 -> Subtract5/2
  Add4/1 -> Multiply4/1
  Abs/1 -> Gain/1
  Sign4/1 -> Subtract4/2
  Sign2/1 -> Subtract2/2
  Subtract6/1 -> fhan/1
  Subtract/1 -> Gain1/1
  Gain3/1 -> Multiply5/3  "sa"
  v2/1 -> Multiply1/1
  Gain2/1 -> Multiply4/2  "sy"
  Sign/1 -> Multiply3/1
  v1/1 -> Add/1

== system old_FMS/Control_Mode/Altitude_Hold_Mode/Command_Generator/Vel_Command/Subsystem1/Height_Control/Position_Error/Bus_Selection ==
  INS_Out : Inport
  Bus Selector2 : BusSelector  OutputSignals=h_R
  Gain : Gain  Gain=-1
  pos_z_O : Outport
  wires:
  Gain/1 -> pos_z_O/1
  Bus Selector2/1 -> Gain/1  "<h_R>"
  INS_Out/1 -> Bus Selector2/1

== system old_FMS/Control_Mode/Altitude_Hold_Mode/Command_Generator/Vel_Command/Subsystem1/Height_Control/Position_Error/Z_Holder ==
  u : Inport
  update : Inport  Port=2
  Delay : Delay  DelayLength=1  InitialConditionSource=Input port
      settings: InputPortMap=u0,p4
  Switch1 : Switch  Criteria=u2 > Threshold
  y : Outport
  wires:
  Switch1/1 -> y/1, Delay/1
  Delay/1 -> Switch1/3
  update/1 -> Switch1/2
  u/1 -> Delay/2, Switch1/1

== system old_FMS/Control_Mode/Position_Mode/Command_Generator/Vel_Command/Subsystem1/Position_Control/Position_Error/Bus_Selection ==
  INS_Out : Inport
  Bus Selector2 : BusSelector  OutputSignals=x_R,y_R,h_R
  Gain : Gain  Gain=-1
  Mux3 : Mux  Inputs=3
  pos_R_O : Outport
  wires:
  Mux3/1 -> pos_R_O/1
  Gain/1 -> Mux3/3
  Bus Selector2/1 -> Mux3/1  "<x_R>"
  Bus Selector2/2 -> Mux3/2  "<y_R>"
  Bus Selector2/3 -> Gain/1  "<h_R>"
  INS_Out/1 -> Bus Selector2/1

== system old_FMS/Control_Mode/Position_Mode/Command_Generator/Vel_Command/Subsystem1/Position_Control/Position_Error/XY_Holder ==
  u : Inport
  update : Inport  Port=2
  Delay : Delay  DelayLength=1  InitialConditionSource=Input port
      settings: InputPortMap=u0,p4
  Switch1 : Switch  Criteria=u2 > Threshold
  y : Outport
  wires:
  u/1 -> Delay/2, Switch1/1
  update/1 -> Switch1/2
  Delay/1 -> Switch1/3
  Switch1/1 -> Delay/1, y/1

== system old_FMS/Control_Mode/Position_Mode/Command_Generator/Vel_Command/Subsystem1/Position_Control/Position_Error/Z_Holder ==
  u : Inport
  update : Inport  Port=2
  Delay : Delay  DelayLength=1  InitialConditionSource=Input port
      settings: InputPortMap=u0,p4
  Switch1 : Switch  Criteria=u2 > Threshold
  y : Outport
  wires:
  Switch1/1 -> y/1, Delay/1
  Delay/1 -> Switch1/3
  update/1 -> Switch1/2
  u/1 -> Delay/2, Switch1/1

== stateflow chart old_FMS/Control_Mode/Mode_Logic ==
  state Unknow
    entry:
    local_mode = 0;
  state Mission
    entry:
    local_mode = 1;
  state Position
    entry:
    local_mode = 2;
  state Altitude_Hold
    entry:
    local_mode = 3;
  state Manual
    entry:
    local_mode = 4;
  state Acro
    entry:
    local_mode = 5;
  (junction 126) -> Unknow
  Unknow -> (junction 130)
  (junction 115) -> (junction 126) [order 2]
  (junction 130) -> (junction 75)
  (junction 115) -> Mission [order 1] : [mode == 1]
  Mission -> (junction 73)
  (junction 73) -> (junction 75) [order 1] : [bitget(flag, 4) && bitget(flag, 6)]
  (junction 50) -> (junction 115) [order 2]
  (junction 73) -> Position [order 2]
  (junction 75) -> (junction 81)
  (junction 50) -> Position [order 1] : [mode == 2]
  Position -> (junction 79)
  (junction 79) -> (junction 81) [order 1] : [bitget(flag, 4) && bitget(flag, 7) && bitget(flag, 8)]
  (junction 53) -> (junction 50) [order 2]
  (junction 79) -> Altitude_Hold [order 2]
  (junction 81) -> (junction 90)
  (junction 53) -> Altitude_Hold [order 1] : [mode == 3]
  Altitude_Hold -> (junction 88)
  (junction 88) -> (junction 90) [order 1] : [bitget(flag, 8)]
  (junction 56) -> (junction 53) [order 2]
  (junction 88) -> Manual [order 2]
  (junction 90) -> (junction 98)
  (junction 56) -> Manual [order 1] : [mode == 4]
  Manual -> (junction 136)
  (junction 136) -> (junction 98) [order 1] : [bitget(flag, 3)]
  (junction 59) -> (junction 56) [order 2]
  (junction 136) -> Acro [order 2]
  (junction 98) -> (junction 103)
  (default) -> (junction 59)
  (junction 59) -> Acro [order 1] : [mode == 5]
  Acro -> (junction 103)
  (junction 108) -> (junction 59)
  (junction 103) -> (junction 106)
  (junction 106) -> (junction 108) : {control_mode = local_mode;}
  data: mode input; local_mode local uint32; flag input uint32; control_mode output

== stateflow chart old_FMS/Control_Mode/Altitude_Hold_Mode/Command_Generator/Psi_Rate_Command/Motion_State ==
  state Hold
    entry:
    state=2;
  state Move
    entry:
    state=0;
  state Brake
    entry:
    state=1;
  (default) -> Move
  Hold -> Move : [move_cmd==1]
  Move -> Brake : [move_cmd==0]
  Brake -> Move [order 2] : [move_cmd==1]
  Brake -> Hold [order 1] : [heading_rate<=0.1 || after(1, sec)]
  data: move_cmd input; heading_rate input; state output

== stateflow chart old_FMS/State_Management/Arm_Event/Arm_Event ==
  state Idle
    en:
    arm_event = 0;
  state arm_event
    en:
    arm_event = 1;
  state ready
  (default) -> Idle
  arm_event -> Idle
  Idle -> ready : [stick_throttle < -0.8 && stick_roll < -0.8 && stick_pitch < -0.8]
  ready -> arm_event : [abs(stick_roll) < 0.15 && abs(stick_pitch)<0.15]
  data: stick_roll input; stick_pitch input; stick_throttle input; arm_event output

== stateflow chart old_FMS/State_Management/State_Logic ==
  state Motor_Test
    entry:
    State = 1;
    during:
    PWM_Cmd = 1000 + uint16((Stick_Throttle+1)*500);
  state Disarm
    entry:
    State = 0;
    PWM_Cmd = 1000;
  state Arm
    entry:
    State = 2;
  state Standby
    entry:
    State = 1;
    PWM_Cmd = 1150;
  Disarm -> Motor_Test [order 1] : [Test_Motor == 1 && Arm_Event == 1]
  Motor_Test -> Disarm : [Test_Motor == 0 || Arm_Event == 1]
  (default) -> Disarm
  Arm -> Disarm [order 1] : [Disarm_Event == 1 && Disarm_Allowed == 1]
  Arm -> Disarm [order 2] : [Force_Disarm]
  Disarm -> Standby [order 2] : [Arm_Event == 1 && Arm_Allowed == 1]
  Standby -> Disarm [order 1] : after(30,sec)
  Standby -> Disarm [order 3] : [Arm_Event == 1 || Force_Disarm]
  Standby -> Arm [order 2] : [Stick_Throttle > -0.25]
  data: PWM_Cmd output uint16; State output; Arm_Allowed input; Disarm_Allowed input; Arm_Event input; Disarm_Event input; Stick_Throttle input; Force_Disarm input; Test_Motor input

== stateflow chart old_FMS/Control_Mode/Manual_Mode/Command_Generator/Psi_Rate_Command/Motion_State ==
  state Hold
    entry:
    state=2;
  state Move
    entry:
    state=0;
  state Brake
    entry:
    state=1;
  (default) -> Move
  Hold -> Move : [move_cmd==1]
  Move -> Brake : [move_cmd==0]
  Brake -> Move [order 2] : [move_cmd==1]
  Brake -> Hold [order 1] : [heading_rate<=0.1 || after(1, sec)]
  data: move_cmd input; heading_rate input; state output

== stateflow chart old_FMS/Control_Mode/Position_Mode/Command_Generator/Vel_Command/Motion_State/XY_Motion_State ==
  state Hold
    entry:
    state=2;
  state Move
    entry:
    state=0;
  state Brake
    entry:
    state=1;
  (default) -> Move
  Hold -> Move : [move_cmd==1]
  Move -> Brake : [move_cmd==0]
  Brake -> Move [order 2] : [move_cmd==1]
  Brake -> Hold [order 1] : [speed<=0.2 || after(2.5, sec)]
  data: move_cmd input; state output; speed input

== stateflow chart old_FMS/Control_Mode/Position_Mode/Command_Generator/Vel_Command/Motion_State/Z_Motion_State ==
  state Hold
    entry:
    state=2;
  state Move
    entry:
    state=0;
  state Brake
    entry:
    state=1;
  (default) -> Move
  Hold -> Move : [move_cmd==1]
  Move -> Brake : [move_cmd==0]
  Brake -> Move [order 2] : [move_cmd==1]
  Brake -> Hold [order 1] : [abs(speed)<=0.2 || after(1.5, sec)]
  data: move_cmd input; state output; speed input

== stateflow chart old_FMS/Control_Mode/Altitude_Hold_Mode/Command_Generator/Vel_Command/Motion_State/Z_Motion_State ==
  state Hold
    entry:
    state=2;
  state Move
    entry:
    state=0;
  state Brake
    entry:
    state=1;
  (default) -> Move
  Hold -> Move : [move_cmd==1]
  Move -> Brake : [move_cmd==0]
  Brake -> Move [order 2] : [move_cmd==1]
  Brake -> Hold [order 1] : [abs(speed)<=0.2 || after(1.5, sec)]
  data: move_cmd input; state output; speed input

== stateflow chart old_FMS/State_Management/Arm_Event/Disarm_Event ==
  state Disarm
    en:
    disarm_event = 1;
  state Idle
    en:
    disarm_event = 0;
  state On_Ground
  (default) -> Idle
  Disarm -> Idle
  On_Ground -> Disarm [order 2] : [after(1.5, sec)]
  On_Ground -> Idle [order 1] : [on_ground == 0]
  Idle -> On_Ground : [on_ground == 1 && state == 2]
  data: on_ground input; disarm_event output; state input

== stateflow chart old_FMS/Control_Mode/Position_Mode/Command_Generator/Psi_Rate_Command1/Motion_State ==
  state Hold
    entry:
    state=2;
  state Move
    entry:
    state=0;
  state Brake
    entry:
    state=1;
  (default) -> Move
  Hold -> Move : [move_cmd==1]
  Move -> Brake : [move_cmd==0]
  Brake -> Move [order 2] : [move_cmd==1]
  Brake -> Hold [order 1] : [heading_rate<=0.1 || after(1, sec)]
  data: move_cmd input; heading_rate input; state output
